simulink model "sensor_acquistion"  (R2023b)
settings: Solver=FixedStepAuto  StartTime=0.0  StopTime=10.0  FixedStep=1e-3  RelTol=1e-3
undefined symbols (not defined in the file): tol_Baro_Alt, tol_GPS, tol_IMU, tol_Mag, tol_Pitot
settings Model: DataDictionary=sensor_datasheet.sldd  PauseTimes=0.1  Creator=Aniket  LastModifiedBy=Aniket
settings ConfigComp: DVTestSuiteOptimization=Auto  DVDetectOutOfBounds=on  DVModelReferenceHarness=on  DVHarnessSource=Signal Editor  DVRebuildModelRepresentation=IfChangeIsDetected

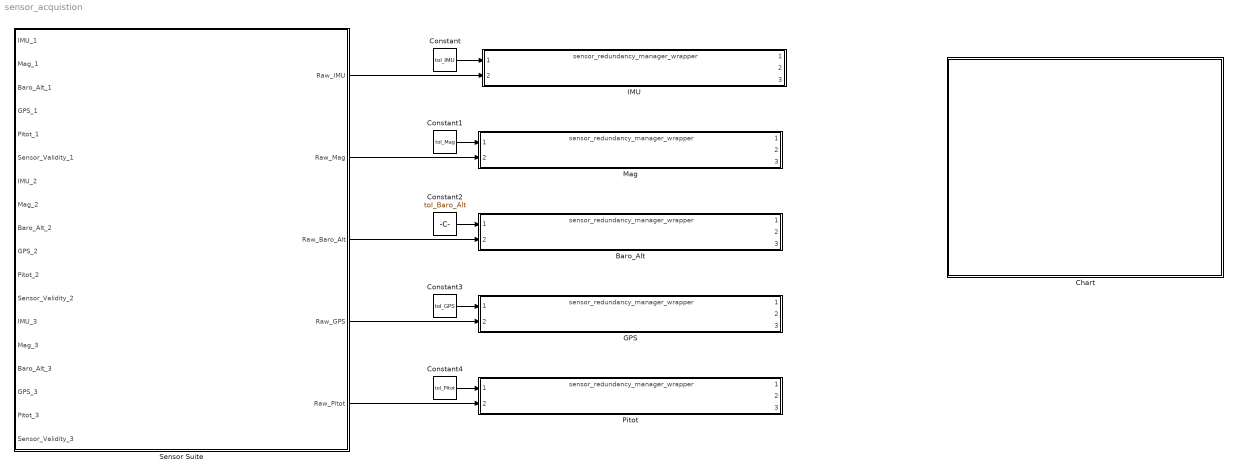
== system sensor_acquistion ==
  Baro_Alt : ModelReference  ModelNameDialog=sensor_redundancy_manager_wrapper.mdl  SimulationMode=Normal  ModelReferenceVersion=1.3
  Chart : Stateflow chart  TreatAsAtomicUnit=on
  Constant : Constant  Value=tol_IMU
  Constant1 : Constant  Value=tol_Mag
  Constant2 : Constant  Value=tol_Baro_Alt
  Constant3 : Constant  Value=tol_GPS
  Constant4 : Constant  Value=tol_Pitot
  GPS : ModelReference  ModelNameDialog=sensor_redundancy_manager_wrapper.mdl  SimulationMode=Normal  ModelReferenceVersion=1.3
  IMU : ModelReference  ModelNameDialog=sensor_redundancy_manager_wrapper.mdl  SimulationMode=Normal  ModelReferenceVersion=1.3
  Mag : ModelReference  ModelNameDialog=sensor_redundancy_manager_wrapper.mdl  SimulationMode=Normal  ModelReferenceVersion=1.3
  Pitot : ModelReference  ModelNameDialog=sensor_redundancy_manager_wrapper.mdl  SimulationMode=Normal  ModelReferenceVersion=1.3
  Sensor Suite : Subsystem
  wires:
  Sensor Suite/1(Raw_IMU) -> IMU/2
  Sensor Suite/2(Raw_Mag) -> Mag/2
  Sensor Suite/3(Raw_Baro_Alt) -> Baro_Alt/2
  Sensor Suite/4(Raw_GPS) -> GPS/2
  Sensor Suite/5(Raw_Pitot) -> Pitot/2
  Constant/1 -> IMU/1
  Constant1/1 -> Mag/1
  Constant2/1 -> Baro_Alt/1
  Constant3/1 -> GPS/1
  Constant4/1 -> Pitot/1

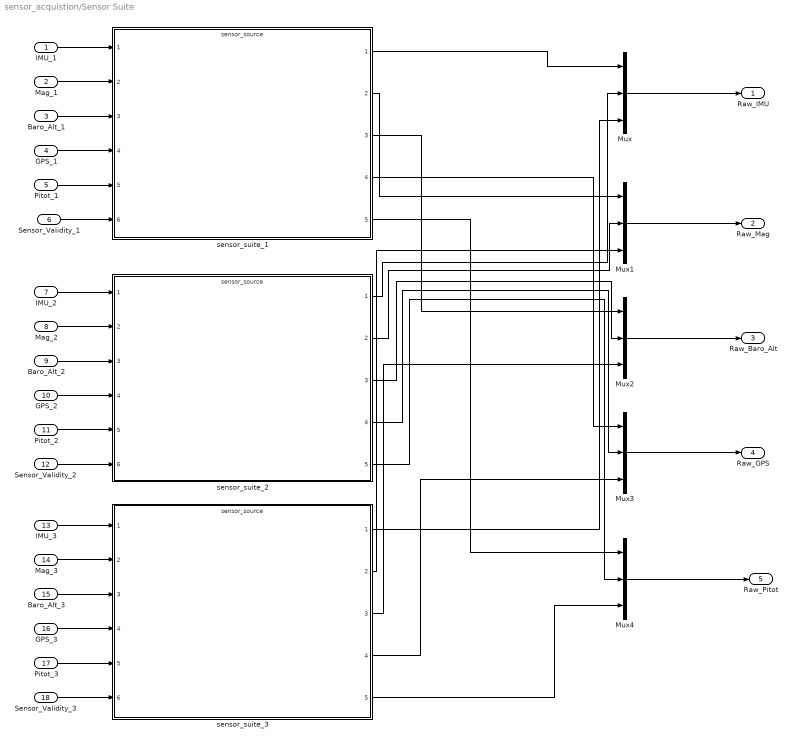
== system sensor_acquistion/Sensor Suite ==
  IMU_1 : Inport
  Mag_1 : Inport  Port=2
  Baro_Alt_1 : Inport  Port=3
  GPS_1 : Inport  Port=4
  Pitot_1 : Inport  Port=5
  Sensor_Validity_1 : Inport  Port=6
  IMU_2 : Inport  Port=7
  Mag_2 : Inport  Port=8
  Baro_Alt_2 : Inport  Port=9
  GPS_2 : Inport  Port=10
  Pitot_2 : Inport  Port=11
  Sensor_Validity_2 : Inport  Port=12
  IMU_3 : Inport  Port=13
  Mag_3 : Inport  Port=14
  Baro_Alt_3 : Inport  Port=15
  GPS_3 : Inport  Port=16
  Pitot_3 : Inport  Port=17
  Sensor_Validity_3 : Inport  Port=18
  Mux{,1..4} (5 alike) : Mux  Inputs=3
  sensor_suite_1 : ModelReference  ModelNameDialog=sensor_source.slx  SimulationMode=Normal  ModelReferenceVersion=1.6
  sensor_suite_2 : ModelReference  ModelNameDialog=sensor_source.slx  SimulationMode=Normal  ModelReferenceVersion=1.6
  sensor_suite_3 : ModelReference  ModelNameDialog=sensor_source.slx  SimulationMode=Normal  ModelReferenceVersion=1.6
  Raw_IMU : Outport
  Raw_Mag : Outport  Port=2
  Raw_Baro_Alt : Outport  Port=3
  Raw_GPS : Outport  Port=4
  Raw_Pitot : Outport  Port=5
  wires:
  IMU_1/1 -> sensor_suite_1/1
  Mag_1/1 -> sensor_suite_1/2
  Baro_Alt_1/1 -> sensor_suite_1/3
  sensor_suite_1/1 -> Mux/1
  GPS_1/1 -> sensor_suite_1/4
  Pitot_1/1 -> sensor_suite_1/5
  IMU_2/1 -> sensor_suite_2/1
  Mag_2/1 -> sensor_suite_2/2
  Mux/1 -> Raw_IMU/1
  Baro_Alt_2/1 -> sensor_suite_2/3
  sensor_suite_1/2 -> Mux1/1
  GPS_2/1 -> sensor_suite_2/4
  Pitot_2/1 -> sensor_suite_2/5
  IMU_3/1 -> sensor_suite_3/1
  Mux2/1 -> Raw_Baro_Alt/1
  Mag_3/1 -> sensor_suite_3/2
  Baro_Alt_3/1 -> sensor_suite_3/3
  GPS_3/1 -> sensor_suite_3/4
  Pitot_3/1 -> sensor_suite_3/5
  sensor_suite_1/3 -> Mux2/1
  sensor_suite_1/4 -> Mux3/1
  sensor_suite_1/5 -> Mux4/1
  sensor_suite_2/1 -> Mux/2
  sensor_suite_2/2 -> Mux1/2
  sensor_suite_2/3 -> Mux2/2
  sensor_suite_2/4 -> Mux3/2
  sensor_suite_2/5 -> Mux4/2
  sensor_suite_3/1 -> Mux/3
  sensor_suite_3/3 -> Mux2/3
  sensor_suite_3/2 -> Mux1/3
  sensor_suite_3/5 -> Mux4/3
  sensor_suite_3/4 -> Mux3/3
  Mux1/1 -> Raw_Mag/1
  Mux3/1 -> Raw_GPS/1
  Mux4/1 -> Raw_Pitot/1
  Sensor_Validity_1/1 -> sensor_suite_1/6
  Sensor_Validity_2/1 -> sensor_suite_2/6
  Sensor_Validity_3/1 -> sensor_suite_3/6

== stateflow chart sensor_acquistion/Chart ==
  state Healthy
  (default) -> Healthy
